simulink model "fsk"  (R2018a)
settings: Solver=VariableStepAuto  StartTime=0.0  StopTime=10  RelTol=1e-3
undefined symbols (not defined in the file or in its folder): fdesignblkfcn, gcbh
libraries: dspfdesign x2, commchan3 x1, simulink x1, commseqgen3 x1
settings Model: Creator=Владимир  LastModifiedBy=Владимир

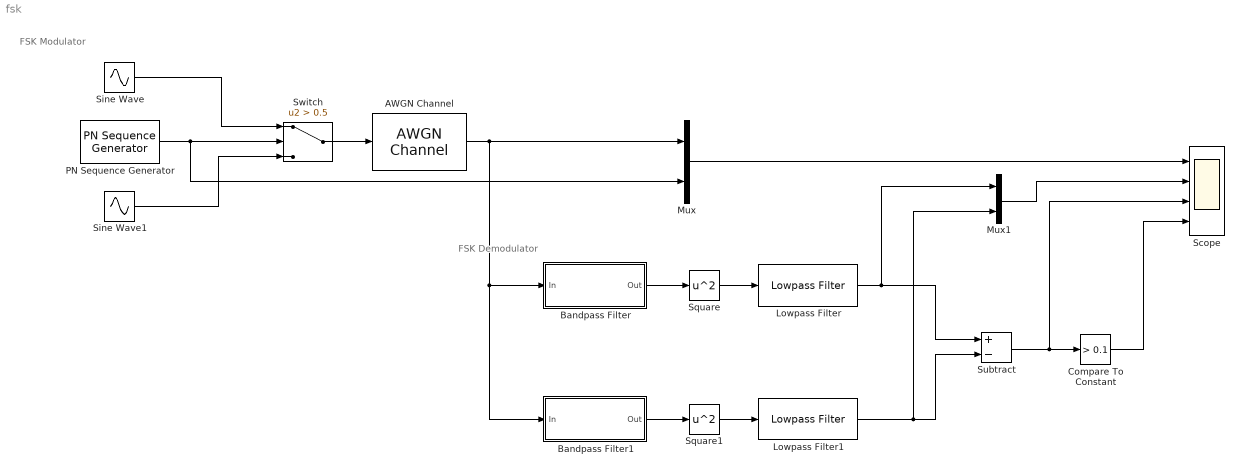
== system fsk ==
  note: FSK Demodulator
  note: FSK Modulator
  AWGN Channel : commchan3/AWGN Channel  InputProcessing=Columns as channels (frame based)  seed=67  noiseMode="Signal to noise ratio  (SNR)"  EbNodB=40  EsNodB=10  SNRdB=30  bitsPerSym=1  Ps=1  Tsym=1  variance=1
  Bandpass Filter : Subsystem  DialogController=fdesignblkfcn  InitFcn=fdesignblkfcn(gcbh, {'InitFcn'});  mask(Bandpass Filter){}
      mask help: Design a bandpass filter
      settings: CopyFcn=fdesignblkfcn(gcbh, {'CopyFcn'});
      mask Help: helpview(mapfilelocation('dsp'), 'dspbandpassfilter');
      mask Display: disp('Bandpass');
  Bandpass Filter1 : Subsystem  DialogController=fdesignblkfcn  InitFcn=fdesignblkfcn(gcbh, {'InitFcn'});  mask(Bandpass Filter){}
      mask help: Design a bandpass filter
      settings: CopyFcn=fdesignblkfcn(gcbh, {'CopyFcn'});
      mask Help: helpview(mapfilelocation('dsp'), 'dspbandpassfilter');
      mask Display: disp('Bandpass');
  Compare To Constant : simulink/Logic and Bit Operations/Compare To Constant  relop=>  const=0.1  OutDataTypeStr=boolean
  Lowpass Filter : dspfdesign/Lowpass Filter  FilterType=FIR  DesignForMinimumOrder=on  FilterOrder=50  PassbandFrequency=5  StopbandFrequency=8  PassbandRipple=1  StopbandAttenuation=60  InheritSampleRate=on  SampleRate=1000  SimulateUsing=Interpreted execution  roundingMode=Floor  coeffsDataTypeStr=fixdt(1,16)
  Lowpass Filter1 : dspfdesign/Lowpass Filter  FilterType=FIR  DesignForMinimumOrder=on  FilterOrder=50  PassbandFrequency=5  StopbandFrequency=8  PassbandRipple=1  StopbandAttenuation=60  InheritSampleRate=on  SampleRate=1000  SimulateUsing=Interpreted execution  roundingMode=Floor  coeffsDataTypeStr=fixdt(1,16)
  Mux : Mux  Inputs=2
  Mux1 : Mux  Inputs=2
  PN Sequence Generator : commseqgen3/PN Sequence Generator  poly='z^6 + z + 1'  ini_sta=[0 1 0 0 0 1]  outBitMaskSource=Dialog parameter  shift=0  outVarSiz=off  maxOutSizeMode=Dialog parameter  maxOutSize=[10 1]  Ts=1  sampPerFrame=1  reset=off  bitPackedOutputs=off  outDataType=double  numPackedBits=8  bitPackDataSigned=off  bitPackedOutDType=double
      settings: SourceProductName=Communications System Toolbox
  Scope : Scope  NumInputPorts=4
  Sine Wave : Sin  Frequency=2*pi*8  Phase=pi/4  SampleTime=0.001
  Sine Wave1 : Sin  Frequency=2*pi*12  Phase=pi/4  SampleTime=0.001
  Square : Math  Operator=square  SaturateOnIntegerOverflow=on
  Square1 : Math  Operator=square  SaturateOnIntegerOverflow=on
  Subtract : Sum  Inputs=+-
  Switch : Switch  Criteria=u2 > Threshold  Threshold=0.5
  wires:
  PN Sequence Generator/1 -> Mux/2, Switch/2
  Switch/1 -> AWGN Channel/1
  Mux/1 -> Scope/1
  Sine Wave/1 -> Switch/1
  Sine Wave1/1 -> Switch/3
  AWGN Channel/1 -> Bandpass Filter/1(In), Bandpass Filter1/1(In), Mux/1
  Lowpass Filter/1 -> Mux1/1, Subtract/1
  Square/1 -> Lowpass Filter/1
  Lowpass Filter1/1 -> Mux1/2, Subtract/2
  Square1/1 -> Lowpass Filter1/1
  Subtract/1 -> Scope/3, Compare To Constant/1
  Bandpass Filter/1(Out) -> Square/1
  Bandpass Filter1/1(Out) -> Square1/1
  Compare To Constant/1 -> Scope/4
  Mux1/1 -> Scope/2

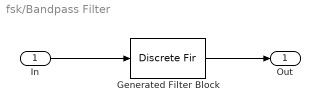
== system fsk/Bandpass Filter ==
  In : Inport
  Generated Filter Block : DiscreteFir  Tag=BlockMethodSubSystem  Coefficients=[-0.000557060532119474524 0.000211453797432160462 0.000182651369273119282 0.000162354068101397539 0.000149190189532817283 0.00014098535827323773 0.000137202616269321604 0.000136286517926051875 0.000138195635253964043 0.000141723543320092975 0.000147134054257652886 0.000153402886730250065 0.000160996168409746924 0.000168960695963061712 0.000177929088053125728 0.000186917612308664478 0.000196770415644801754 0.000206242565531635663 0.000216900480353357039 0.00022608799635077156 0.000237329482122800224 0.000247304304859121186 0.000256883472798200832 0.000267384882670586754 0.000277722346583436424 0.000287429900409670721 0.000296729494568636395 0.000305885349820244484 0.000315058880764832708 0.000323912862481612698 0.000332370789738621196 0.000340161924115166617 0.0003474715700161864 0.00035420970125758745 0.000360558426869292436 0.000366383856512686966 0.000371647430352719621 0.00037632121560775137 0.000380140117585084413 0.000383221337862482995 0.000385696219668682863 0.000386840147923478916 0.000387795337858941693 0.000387595332537656718 0.000386662881820129306 0.000384674544346972605 0.00038216024656221551 0.000378442642104268295 0.000373888498325872654 0.000368077262206721633 0.000361555354701117168 0.000353846104016092397 0.000345353209857500584 0.000335568550883419674 0.000325012006665385865 0.000313242746374552909 0.000300808758011930633 0.000287210085280361423 0.000272816805916949114 0.000257397749031893939 0.00024099964241572824 0.000223692087249350484 0.000205653737798278937 0.000186536813869443035 0.00016680853638125436 0.000146176314331795975 0.0001248830348638708 0.000102660536782754066 7.99639232219065367e-05 5.65402436351833144e-05 3.27127429756169643e-05 8.20172877970975524e-06 -1.65907389906477841e-05 -4.18982304966106873e-05 -6.73694920815492938e-05 -9.33063062593238136e-05 -0.000119281056081081346 -0.000145627278943255274 -0.000171739924249783224 -0.000198094546186803255 -0.000224141707733103426 -0.000250196295067401449 -0.000275940525408778568 -0.000301523622560319208 -0.000326538210117146037 -0.000351294021521197735 -0.000375396167996294781 -0.000399033871231595574 -0.000421847172016398563 -0.000444088098850627913 -0.000465360120938991951 -0.000485850337562336121 -0.000505222393275927498 -0.000523721168924530609 -0.000541041259488000449 -0.00055731869242771348 -0.000572289349517980661 -0.000586068167209887348 -0.000598429405186772087 -0.000609561534748238854 -0.000619080245371525549 -0.000627307920019631784 -0.000633874731562370126 -0.000639028754338299108 -0.000642501550663151545 -0.000644525304798190769 -0.000644751737102193566 -0.000643470182403352775 -0.000640422565568719328 -0.000635870154638360028 -0.000629513812666527769 -0.000621652575609102256 -0.000612006032121420549 -0.000600868495356676855 -0.00058793475025876714 -0.000573556131647923488 -0.000557477343827419243 -0.000539991917871924815 -0.000520909681228195988 -0.000500443671072065043 -0.00047849206016676221 -0.000455325561465024181 -0.0004307493146709685 -0.000405075607405078729 -0.000378139290514334749 -0.000350211591600802213 -0.000321170748902407824 -0.000291330265665551858 -0.000260535207220127882 -0.000229078353563729581 -0.00019686646565424148 -0.000164202826964290568 -0.000130964686627602772 -9.74365692937525542e-05 -6.35186816073631455e-05 -2.95430375203180546e-05 4.64626329923210381e-06 3.86634725525378774e-05 7.268129924892328e-05 0.000106323986345466964 0.000139726031823941333 0.00017259579225457108 0.000205029174295229635 0.000236683943763339299 0.00026770185528809335 0.000297758916988041886 0.000326977574950778065 0.000355060812446438934 0.000382139147278371663 0.000407886644286760544 0.000432443915531716973 0.000455534600450719588 0.000477290921120966346 0.000497433570861372963 0.00051607599577022014 0.00053301022500183736 0.000548338075009643672 0.000561841442705651424 0.000573668285464539319 0.000583575709096187389 0.000591764800417436047 0.000597999048242249596 0.000602450055108387289 0.000604934003642023429 ...(+19686 chars)]  InputProcessing=Columns as channels (frame based)
  Out : Outport
  wires:
  In/1 -> Generated Filter Block/1
  Generated Filter Block/1 -> Out/1

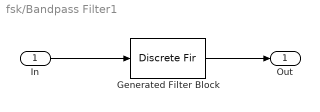
== system fsk/Bandpass Filter1 ==
  In : Inport
  Generated Filter Block : DiscreteFir  Tag=BlockMethodSubSystem  Coefficients=[0.00910480466180604853 -0.00122231453089864314 -0.00113872601553866026 -0.00107450965954138285 -0.00100261564092619937 -0.000949203203456098349 -0.00088710989854036415 -0.000842768955368920075 -0.000788751956436989365 -0.000751945401784828021 -0.000704432249374694133 -0.000673879161302888205 -0.000631424864500122751 -0.00060615027623723769 -0.000567243234781659653 -0.000547151579641668925 -0.000506755346268530568 -0.000501656286901172588 -0.000455374156928391866 -0.000435454239407996949 -0.000416626412293738882 -0.000401194401784703281 -0.000373423241327497379 -0.000354184000984495914 -0.000326289355777303891 -0.000310854748597353542 -0.00028667967438322263 -0.000274612516236213966 -0.000251808914450988089 -0.000240402151725573748 -0.000216992079320941361 -0.000205577168447709097 -0.000181372711444539522 -0.00017184728947944837 -0.000146883091636764579 -0.000138731353137768604 -0.000120900934844944685 -0.00010928827981404772 -9.24280674573889349e-05 -8.76624259013945167e-05 -7.35789115909983582e-05 -6.93129123878893916e-05 -5.52160229106649775e-05 -5.27512091576132908e-05 -4.13888627836273698e-05 -4.21740438068286816e-05 -3.32975602103172119e-05 -3.62189630017349662e-05 -2.88520145738154626e-05 -3.39064907853899727e-05 -2.83891436100615346e-05 -3.62792387614135903e-05 -3.46173896895955041e-05 -4.30988090103154309e-05 -4.57347145881165096e-05 -5.7630511028243514e-05 -5.95929597230916014e-05 -7.27319844424229034e-05 -7.68814934001601363e-05 -9.14911987251066511e-05 -9.55536319014269747e-05 -0.000109762442660785858 -0.000113695374419034434 -0.000128235481277102353 -0.000132170660960474751 -0.000146069518364357054 -0.000148386426331074961 -0.000160169158091293465 -0.000160332072133881343 -0.000168889301362001518 -0.000167556095886240916 -0.000172998891103288976 -0.000167464653633302846 -0.000170705543672714649 -0.000161397861096314668 -0.000159628959904465142 -0.000145739669461590962 -0.00014015344552686243 -0.000122191900953820889 -0.000111822001164932003 -8.86882335024187507e-05 -7.32732955626442389e-05 -4.54057441226386055e-05 -2.5272955407447395e-05 7.31616935864196072e-06 3.26663347144789951e-05 6.95449649498729866e-05 9.95891255349875409e-05 0.000140308362245978452 0.000172613312802195884 0.000216701569009273426 0.000251565366502786922 0.000296986921133715262 0.000333226019230846784 0.000379980302237079362 0.000416635539166996041 0.000462521288367002611 0.000497605025651109631 0.000541477298181186617 0.000574154392383804599 0.000614659001000045571 0.000643170740721716802 0.000678296243965358439 0.000701204170515223879 0.00072984051324942803 0.000745319335333715152 0.000766637580449576125 0.000773113241730570208 0.000784730508820765879 0.000781775445471952907 0.000783180831708642569 0.000769235615527134528 0.00075939024217381787 0.000734202949101878458 0.00071254933191518266 0.000675070223098780606 0.000640829257496759036 0.000591137145063607219 0.00054484500493050779 0.00048349722958334132 0.000425452590080539761 0.000352544414591189278 0.0002838032711882741 0.000200174185331289389 0.000121749392982985552 2.9385520103094101e-05 -5.7755811078292682e-05 -0.000157756527377216765 -0.000251219484318535372 -0.000356491214446559915 -0.000454420695247068768 -0.000562754305338026076 -0.000662372432565292227 -0.00077101391504794288 -0.00086985748223937856 -0.000976215119247423463 -0.00107121723347015918 -0.00117201748023836906 -0.00125980313895575173 -0.00135241389890619103 -0.00143031298089594389 -0.00151160268574007314 -0.00157708655133850621 -0.00164394074669704446 -0.00169375510751545826 -0.00174394978966954314 -0.00177589936548961172 -0.00180673816667431889 -0.00181844010777561411 -0.00182820640039593578 -0.00181809313250740762 -0.0018051710827830976 -0.00177188793903249216 -0.00173548140557213369 -0.00167843666834936733 -0.00161818105836655443 -0.00153694270809183985 -0.00145277634976100252 -0.00134829946966388836 -0.0012410677776830345 -0.00111459147514496489 -0.000986093090524059121 -0.000839073240489675992 ...(+13017 chars)]  InputProcessing=Columns as channels (frame based)
  Out : Outport
  wires:
  In/1 -> Generated Filter Block/1
  Generated Filter Block/1 -> Out/1
